simulink model "uz_mpc_6ph"  (R2021a)
settings: Solver=FixedStepDiscrete  StartTime=0.0  StopTime=3*1/f  RelTol=1e-3
values from neighbouring files (symbols this model uses):
  A = 1.0    (= 1)    [uz_6ph_pu_vsd_voltages_init.m]    (also in uz_mpc_6ph_init.m; uz_mpc_6ph_state_machine_init.m = 0.1)
  f = n_rpm/60.0*p    (= 250)    [uz_6ph_pu_vsd_voltages_init.m]    (also in uz_mpc_6ph_init.m; uz_mpc_6ph_state_machine_init.m = 83.3333333333)
  IB = sqrt(2)*IR    [uz_6ph_pu_vsd_voltages_init.m]    (also in uz_mpc_6ph_init.m; uz_mpc_6ph_state_machine_init.m)
  id_ref = 0.0    (= 0)    [uz_6ph_pu_vsd_voltages_init.m]    (also in uz_mpc_6ph_init.m; uz_mpc_6ph_state_machine_init.m)
  iq_ref = -10.0    (= -10)    [uz_6ph_pu_vsd_voltages_init.m]    (also in uz_mpc_6ph_init.m; uz_mpc_6ph_state_machine_init.m = 5)
  ix_ref = 0.0    (= 0)    [uz_6ph_pu_vsd_voltages_init.m]    (also in uz_mpc_6ph_init.m; uz_mpc_6ph_state_machine_init.m)
  iy_ref = 0.0    (= 0)    [uz_6ph_pu_vsd_voltages_init.m]    (also in uz_mpc_6ph_init.m; uz_mpc_6ph_state_machine_init.m)
  Ld_minus_Lq_over_LB = (Ld-Lq)/LB    [uz_6ph_pu_vsd_voltages_init.m]    (also in uz_mpc_6ph_init.m; uz_mpc_6ph_state_machine_init.m)
  Ld_over_LB = Ld/LB    [uz_6ph_pu_vsd_voltages_init.m]    (also in uz_mpc_6ph_init.m; uz_mpc_6ph_state_machine_init.m)
  Lq_over_LB = Lq/LB    [uz_6ph_pu_vsd_voltages_init.m]    (also in uz_mpc_6ph_init.m; uz_mpc_6ph_state_machine_init.m)
  omega_m = n_rpm*pi/30    (= 314.159265359)    [uz_6ph_pu_vsd_voltages_init.m]    (also in uz_mpc_6ph_init.m; uz_mpc_6ph_state_machine_init.m = 104.71975512)
  omegaB = nR*2*pi()/60*p    [uz_6ph_pu_vsd_voltages_init.m]    (also in uz_mpc_6ph_init.m; uz_mpc_6ph_state_machine_init.m)
  psi_pm_over_psiB = psi_pm/psiB    [uz_6ph_pu_vsd_voltages_init.m]    (also in uz_mpc_6ph_init.m; uz_mpc_6ph_state_machine_init.m)
  Rs_over_ZB = Rs/ZB    [uz_6ph_pu_vsd_voltages_init.m]    (also in uz_mpc_6ph_init.m; uz_mpc_6ph_state_machine_init.m)
  t_ADC = 1/f_ADC    (= 1e-05)    [uz_6ph_pu_vsd_voltages_init.m]    (also in uz_mpc_6ph_init.m; uz_mpc_6ph_state_machine_init.m; uz_typeconv_init.m)
  Ts_times_ZB_over_Ld = Ts*ZB/Ld    [uz_6ph_pu_vsd_voltages_init.m]    (also in uz_mpc_6ph_init.m; uz_mpc_6ph_state_machine_init.m)
  Ts_times_ZB_over_Lq = Ts*ZB/Lq    [uz_6ph_pu_vsd_voltages_init.m]    (also in uz_mpc_6ph_init.m; uz_mpc_6ph_state_machine_init.m)
  Ts_times_ZB_over_Lx = Ts*ZB/Lx    [uz_6ph_pu_vsd_voltages_init.m]    (also in uz_mpc_6ph_init.m; uz_mpc_6ph_state_machine_init.m)
  Ts_times_ZB_over_Ly = Ts*ZB/Ly    [uz_6ph_pu_vsd_voltages_init.m]    (also in uz_mpc_6ph_init.m; uz_mpc_6ph_state_machine_init.m)
  v_dc = 565.0    (= 565)    [uz_6ph_pu_vsd_voltages_init.m]    (also in uz_mpc_6ph_init.m; uz_mpc_6ph_state_machine_init.m)
  VB = sqrt(2/3)*VR    [uz_6ph_pu_vsd_voltages_init.m]    (also in uz_mpc_6ph_init.m; uz_mpc_6ph_state_machine_init.m)
libraries: fl_lib x7, nesl_utility x7, simulink x4, ee_lib x2, hdlsllib x1
(part 2 of 2)

== matlab function uz_mpc_6ph/error_calculation ==
  settings: fimath=fimath('RoundingMethod', 'Floor','OverflowAction', 'Wrap','ProductMode', 'FullPrecision', 'SumMode', 'FullPrecision')
  data: id_ref_pu input; e_id_pu output; iq_ref_pu input; ix_ref_pu input; iy_ref_pu input; id_pred_pu input; iq_pred_pu input; ix_pred_pu input; iy_pred_pu input; max_current_pu input; G input; e_iq_pu output; e_ix_pu output; e_iy_pu output; delta_u output; index_prev input
function [e_id_pu, e_iq_pu, e_ix_pu, e_iy_pu, delta_u] = error_calculation(id_ref_pu,iq_ref_pu,ix_ref_pu,iy_ref_pu,id_pred_pu,iq_pred_pu,ix_pred_pu,iy_pred_pu,max_current_pu,G, index_prev)

num_switching_states = 64;

fm = fimath();
id_ref_pu = fi(id_ref_pu,1,18,15,fm);
iq_ref_pu = fi(iq_ref_pu,1,18,15,fm);
ix_ref_pu = fi(ix_ref_pu,1,18,15,fm);
iy_ref_pu = fi(iy_ref_pu,1,18,15,fm);

id_pred_pu = fi(zeros(num_switching_states,1),1,27,24,fm);
iq_pred_pu = fi(zeros(num_switching_states,1),1,27,24,fm);
ix_pred_pu = fi(zeros(num_switching_states,1),1,27,24,fm);
iy_pred_pu = fi(zeros(num_switching_states,1),1,27,24,fm);

max_current_pu = fi(max_current_pu,1,18,15,fm);

e_id_pu = fi(zeros(num_switching_states,1),1,18,15,fm);
e_iq_pu = fi(zeros(num_switching_states,1),1,18,15,fm);
e_ix_pu = fi(zeros(num_switching_states,1),1,18,15,fm);
e_iy_pu = fi(zeros(num_switching_states,1),1,18,15,fm);
d_u = fi(zeros(num_switching_states,6),0,18,0,fm);


for i=1:num_switching_states %(SZ+1) für die 4 Schalterstellungen im ersten Zeithorizont den Fehler berechnen
    e_id_pu(i) = (id_ref_pu-id_pred_pu(i))^2;
    e_iq_pu(i) = (iq_ref_pu-iq_pred_pu(i))^2;
    e_ix_pu(i) = (ix_ref_pu-ix_pred_pu(i))^2;
    e_iy_pu(i) = (iy_ref_pu-iy_pred_pu(i))^2;
    % check for current limit
    check_limit = fi(sqrt(id_pred_pu(i)^2+iq_pred_pu(i)^2+ix_pred_pu(i)^2+iy_pred_pu(i)^2),1,18,15,fm);
    if ( check_limit > max_current_pu)
        e_id_pu(i) = 3.99; % max value for Sfix18_En15
        e_iq_pu(i) = 3.99;
        e_ix_pu(i) = 3.99;
        e_iy_pu(i) = 3.99;
    end
    % calculate switching effort
    G_next = [G(i,1), G(i,3), G(i,5), G(i,7), G(i,9), G(i,11)];
    G_prev = [G(index_prev,1), G(index_prev,3), G(index_prev,5), G(index_prev,7), G(index_prev,9), G(index_prev,11)];
    d_u(i,:) = (G_prev -  G_next).^2;
end


delta_u = fi(sum(d_u,2),0,18,0,fm); % Summe jeder Zeile von d_u, um die Summe an Umschaltvorgängen zu erhalten
end

== matlab function uz_mpc_6ph/cost_function ==
  settings: fimath=fimath('RoundingMethod', 'Floor','OverflowAction', 'Wrap','ProductMode', 'FullPrecision', 'SumMode', 'FullPrecision')
  data: e_id_pu input; costs output; e_iq_pu input; e_ix_pu input; e_iy_pu input; delta_u input; lambda_d input; lambda_q input; lambda_x input; lambda_y input; lambda_u input
function costs = cost_function(e_id_pu,e_iq_pu,e_ix_pu,e_iy_pu,delta_u,lambda_d,lambda_q,lambda_x,lambda_y,lambda_u)

fm = fimath();
lambda_d = fi(lambda_d,0,18,17,fm);
lambda_q = fi(lambda_q,0,18,17,fm);
lambda_x = fi(lambda_x,0,18,17,fm);
lambda_y = fi(lambda_y,0,18,17,fm);
lambda_u = fi(lambda_u,0,18,17,fm);

% error could be worst case 4^2 for each current component + 12^2 for
% switching effort = 208. Fits into sfix27_En18
costs = fi(lambda_d * e_id_pu + lambda_q * e_iq_pu + lambda_x * e_ix_pu + lambda_y * e_iy_pu + lambda_u * delta_u,1,27,18,fm);

end

== matlab function uz_mpc_6ph/MATLAB Function ==
  settings: fimath=fimath('RoundingMethod', 'Floor','OverflowAction', 'Wrap','ProductMode', 'FullPrecision', 'SumMode', 'FullPrecision')
  data: costs input; id_pred_pu input; iq_pred_pu input; ix_pred_pu input; iy_pred_pu input; index output; id_pred_idx_pu output; iq_pred_idx_pu output; ix_pred_idx_pu output; iy_pred_idx_pu output; G input; Gates output
function [index, id_pred_idx_pu, iq_pred_idx_pu, ix_pred_idx_pu, iy_pred_idx_pu, Gates] = optimize_costs(costs, id_pred_pu, iq_pred_pu, ix_pred_pu,iy_pred_pu, G)

fm = fimath();
costs = fi(costs,1,27,18,fm);


[m, idx] = min(costs);
index = fi(idx,0,18,0,fm);
Gates = [G(index,1),G(index,2),G(index,3),G(index,4),G(index,5),G(index,6),...
         G(index,7),G(index,8),G(index,9),G(index,10),G(index,11),G(index,12)]; 
id_pred_idx_pu = id_pred_pu(index);
iq_pred_idx_pu = iq_pred_pu(index);
ix_pred_idx_pu = ix_pred_pu(index);
iy_pred_idx_pu = iy_pred_pu(index);

end

== matlab function uz_mpc_6ph/uz_mpc_current ==
  data: id_pu input fixdt_type_dq_currents; iq_pu input fixdt_type_dq_currents; ix_pu input fixdt_type_xy_currents; iy_pu input fixdt_type_xy_currents; angle_el input fixdt_type_angle; vd_pu input fixdt_type_sin_cos; vq_pu input fixdt_type_sin_cos; vx_pu input; vy_pu input; omega_pu input fixdt_type_speed; id_ref_pu input fixdt_type_dqxy_ref_currents; iq_ref_pu input fixdt_type_dqxy_ref_currents; ix_ref_pu input fixdt_type_dqxy_ref_currents; iy_ref_pu input fixdt_type_dqxy_ref_currents; v_DC_pu input fixdt_type_voltage; G output boolean; i_d_pred_pu output fixdt_type_dqxy_ref_currents; i_q_pred_pu output fixdt_type_dqxy_ref_currents; i_x_pred_pu output fixdt_type_dqxy_ref_currents; i_y_pred_pu output fixdt_type_dqxy_ref_currents; T_el_pred_pu output fixdt_type_dqxy_ref_currents; index output fixdt_type_polepairs; id_delay_pu output fixdt_type_dqxy_ref_currents; iq_delay_pu output fixdt_type_dqxy_ref_currents; Rs_over_ZB input fixdt_type_constants; Ts_times_ZB_over_Ld input fixdt_type_constants; Ts_times_ZB_over_Lq input fixdt_type_constants; Ts_times_ZB_over_Lx input fixdt_type_constants; Ts_times_ZB_over_Ly input fixdt_type_constants; Ld_over_LB input fixdt_type_constants; Lq_over_LB input fixdt_type_constants; Ld_minus_Lq_over_LB input fixdt_type_constants; psi_pm_over_psiB input fixdt_type_constants; polepairs input fixdt_type_polepairs; max_current_pu input fixdt_type_max_current; lambda_u input fixdt_type_lambda; lambda_d input fixdt_type_lambda; lambda_q input fixdt_type_lambda; lambda_x input fixdt_type_lambda; lambda_y input fixdt_type_lambda
function [G,i_d_pred_pu,i_q_pred_pu,i_x_pred_pu,i_y_pred_pu,T_el_pred_pu,index,id_delay_pu,iq_delay_pu] = myMPC(id_pu,iq_pu,ix_pu,iy_pu,angle_el,vd_pu,vq_pu,vx_pu,vy_pu,omega_pu, id_ref_pu,iq_ref_pu,ix_ref_pu,iy_ref_pu, v_DC_pu, Rs_over_ZB, Ts_times_ZB_over_Ld, Ts_times_ZB_over_Lq, Ts_times_ZB_over_Lx, Ts_times_ZB_over_Ly, Ld_over_LB, Lq_over_LB, Ld_minus_Lq_over_LB, psi_pm_over_psiB, polepairs, max_current_pu, lambda_u, lambda_d, lambda_q, lambda_x, lambda_y)

% previous index of switching states
persistent index_prev; 
    if isempty(index_prev)
        index_prev = 1;
    end
    
    
    
    
    
    num_switching_states=64;   %Schalterzustände
    ui16_n=1;    %Position in der Fehlermatrix


    persistent G_prev;
    
    if isempty(G_prev)
        G_prev = boolean([0 0 0 0 0 0]);
    end
    
    e_iq = zeros(num_switching_states,1);
    e_id = zeros(num_switching_states,1);
    e_ix = zeros(num_switching_states,1);
    e_iy = zeros(num_switching_states,1);
    delta_u = zeros(num_switching_states,6);
    




    %  V0 V1 V2 V3 V4 V5 V6 V7 V8 V9 V10 V11 V12 V13 V14 V15 V16 V17 V18 V19 V20 V21 V22 V23 V24 V25 V26 V27 V28 V29 V30 V31 V32 V33 V34 V35 V36 V37 V38 V39 V40 V41 V42 V43 V44 V45 V46 V47 V48 V49 V50 V51 V52 V53 V54 V55 V56 V57 V58 V59 V60 V61 V62 V63      (Spannungsvektor)
s1_v = [0; 1; 0; 1; 0; 1; 0; 1; 0; 1; 0; 1; 0; 1; 0; 1; 0; 1; 0; 1; 0; ...
        1; 0; 1; 0; 1; 0; 1; 0; 1; 0; 1; 0; 1; 0; 1; 0; 1; 0; 1; 0; 1; ...
        0; 1; 0; 1; 0; 1; 0; 1; 0; 1; 0; 1; 0; 1; 0; 1; 0; 1; 0; 1; 0; ...
        1];

s2_v = [1; 0; 1; 0; 1; 0; 1; 0; 1; 0; 1; 0; 1; 0; 1; 0; 1; 0; 1; 0; 1; ...
        0; 1; 0; 1; 0; 1; 0; 1; 0; 1; 0; 1; 0; 1; 0; 1; 0; 1; 0; 1; 0; ...
        1; 0; 1; 0; 1; 0; 1; 0; 1; 0; 1; 0; 1; 0; 1; 0; 1; 0; 1; 0; 1; ...
        0];

s3_v = [0; 0; 1; 1; 0; 0; 1; 1; 0; 0; 1; 1; 0; 0; 1; 1; 0; 0; 1; 1; 0; ...
        0; 1; 1; 0; 0; 1; 1; 0; 0; 1; 1; 0; 0; 1; 1; 0; 0; 1; 1; 0; 0; ...
        1; 1; 0; 0; 1; 1; 0; 0; 1; 1; 0; 0; 1; 1; 0; 0; 1; 1; 0; 0; 1; ...
        1];

s4_v = [1; 1; 0; 0; 1; 1; 0; 0; 1; 1; 0; 0; 1; 1; 0; 0; 1; 1; 0; 0; 1; ...
        1; 0; 0; 1; 1; 0; 0; 1; 1; 0; 0; 1; 1; 0; 0; 1; 1; 0; 0; 1; 1; ...
        0; 0; 1; 1; 0; 0; 1; 1; 0; 0; 1; 1; 0; 0; 1; 1; 0; 0; 1; 1; 0; ...
        0];

s5_v = [0; 0; 0; 0; 1; 1; 1; 1; 0; 0; 0; 0; 1; 1; 1; 1; 0; 0; 0; 0; 1; ...
        1; 1; 1; 0; 0; 0; 0; 1; 1; 1; 1; 0; 0; 0; 0; 1; 1; 1; 1; 0; 0; ...
        0; 0; 1; 1; 1; 1; 0; 0; 0; 0; 1; 1; 1; 1; 0; 0; 0; 0; 1; 1; 1; ...
        1];

s6_v = [1; 1; 1; 1; 0; 0; 0; 0; 1; 1; 1; 1; 0; 0; 0; 0; 1; 1; 1; 1; 0; ...
        0; 0; 0; 1; 1; 1; 1; 0; 0; 0; 0; 1; 1; 1; 1; 0; 0; 0; 0; 1; 1; ...
        1; 1; 0; 0; 0; 0; 1; 1; 1; 1; 0; 0; 0; 0; 1; 1; 1; 1; 0; 0; 0; ...
        0];

s7_v = [0; 0; 0; 0; 0; 0; 0; 0; 1; 1; 1; 1; 1; 1; 1; 1; 0; 0; 0; 0; 0; ...
        0; 0; 0; 1; 1; 1; 1; 1; 1; 1; 1; 0; 0; 0; 0; 0; 0; 0; 0; 1; 1; ...
        1; 1; 1; 1; 1; 1; 0; 0; 0; 0; 0; 0; 0; 0; 1; 1; 1; 1; 1; 1; 1; ...
        1];

s8_v = [1; 1; 1; 1; 1; 1; 1; 1; 0; 0; 0; 0; 0; 0; 0; 0; 1; 1; 1; 1; 1; ...
        1; 1; 1; 0; 0; 0; 0; 0; 0; 0; 0; 1; 1; 1; 1; 1; 1; 1; 1; 0; 0; ...
        0; 0; 0; 0; 0; 0; 1; 1; 1; 1; 1; 1; 1; 1; 0; 0; 0; 0; 0; 0; 0; ...
        0];

s9_v = [0; 0; 0; 0; 0; 0; 0; 0; 0; 0; 0; 0; 0; 0; 0; 0; 1; 1; 1; 1; 1; ...
        1; 1; 1; 1; 1; 1; 1; 1; 1; 1; 1; 0; 0; 0; 0; 0; 0; 0; 0; 0; 0; ...
        0; 0; 0; 0; 0; 0; 1; 1; 1; 1; 1; 1; 1; 1; 1; 1; 1; 1; 1; 1; 1; ...
        1];

s10_v = [1; 1; 1; 1; 1; 1; 1; 1; 1; 1; 1; 1; 1; 1; 1; 1; 0; 0; 0; 0; 0; ...
         0; 0; 0; 0; 0; 0; 0; 0; 0; 0; 0; 1; 1; 1; 1; 1; 1; 1; 1; 1; 1; ...
         1; 1; 1; 1; 1; 1; 0; 0; 0; 0; 0; 0; 0; 0; 0; 0; 0; 0; 0; 0; 0; ...
         0];

s11_v = [0; 0; 0; 0; 0; 0; 0; 0; 0; 0; 0; 0; 0; 0; 0; 0; 0; 0; 0; 0; 0; ...
         0; 0; 0; 0; 0; 0; 0; 0; 0; 0; 0; 1; 1; 1; 1; 1; 1; 1; 1; 1; 1; ...
         1; 1; 1; 1; 1; 1; 1; 1; 1; 1; 1; 1; 1; 1; 1; 1; 1; 1; 1; 1; 1; ...
         1];

s12_v = [1; 1; 1; 1; 1; 1; 1; 1; 1; 1; 1; 1; 1; 1; 1; 1; 1; 1; 1; 1; 1; ...
         1; 1; 1; 1; 1; 1; 1; 1; 1; 1; 1; 0; 0; 0; 0; 0; 0; 0; 0; 0; 0; ...
         0; 0; 0; 0; 0; 0; 0; 0; 0; 0; 0; 0; 0; 0; 0; 0; 0; 0; 0; 0; 0; ...
         0];

                          

                
%Berechnung des aktuellen Modells zum Zeitpunkt (k+1), wenn die neue
%Schalterstellung angelegt wird. Dies geschieht anhand der alten,
%vorhergehenden Schalterstellung "idx_alt". Hierdurch wird die Delay-Time
%von einem diskreten Zeitschritt kompensiert!
    [id_delay_pu,iq_delay_pu,ix_delay_pu,iy_delay_pu] = predict_currents(vd_pu(index_prev),vq_pu(index_prev),vx_pu(index_prev),vy_pu(index_prev),id_pu,iq_pu,ix_pu,iy_pu,omega_pu,Ts_times_ZB_over_Ld,Ts_times_ZB_over_Lq,Ts_times_ZB_over_Lx,Ts_times_ZB_over_Ly,Rs_over_ZB,Ld_over_LB,Lq_over_LB,Ld_minus_Lq_over_LB,psi_pm_over_psiB,polepairs);

% id_delay_pu = id_delay_pu;
% iq_delay_pu = iq_delay_pu;
% hier könnte noch Algorithmik zur Eingrenzung der betrachteten
% Schalthandlungen stehen
    

%start Prädiktion %%%%%%%%%%%%%%%%%%%%%%%%%%%%%%%%%%%%%%%%%%%%%%%%%%%%%%%%%%%%%%%
    id_pu_nxt = zeros(num_switching_states, 1);
    iq_pu_nxt = zeros(num_switching_states, 1);
    ix_pu_nxt = zeros(num_switching_states, 1);
    iy_pu_nxt = zeros(num_switching_states, 1);
    T_el_pu_nxt = zeros(num_switching_states, 1);

        

    %Erster Zeithorizont
    for i = 1:num_switching_states
        [id_pu_nxt(i),iq_pu_nxt(i),ix_pu_nxt(i),iy_pu_nxt(i), T_el_pu_nxt(i)] = predict_currents(vd_pu(i),vq_pu(i),vx_pu(i),vy_pu(i),id_delay_pu,iq_delay_pu,ix_delay_pu,iy_delay_pu, omega_pu,Ts_times_ZB_over_Ld,Ts_times_ZB_over_Lq,Ts_times_ZB_over_Lx,Ts_times_ZB_over_Ly,Rs_over_ZB,Ld_over_LB,Lq_over_LB,Ld_minus_Lq_over_LB,psi_pm_over_psiB,polepairs);
    end
    
%end Prädiktion %%%%%%%%%%%%%%%%%%%%%%%%%%%%%%%%%%%%%%%%%%%%%%%%%%%%%%%%%%%



%start Optimierung des Gütekriteriums%%%%%%%%%%%%%%%%%%%%%%%%%%%%%%%%%%%%%%

           for i=1:num_switching_states %(SZ+1) für die 4 Schalterstellungen im ersten Zeithorizont den Fehler berechnen                  
                     e_iq(ui16_n) = (iq_ref_pu-fi(iq_pu_nxt(i),1,18,15))^2;                 
                     e_id(ui16_n) = (id_ref_pu-fi(id_pu_nxt(i),1,18,15))^2;
                     e_ix(ui16_n) = (ix_ref_pu-fi(ix_pu_nxt(i),1,18,15))^2;
                     e_iy(ui16_n) = (iy_ref_pu-fi(iy_pu_nxt(i),1,18,15))^2;
                     % Stromgrenze einhalten
%                      if ( (sqrt(id_pu_nxt(i)^2+iq_pu_nxt(i)^2+ix_pu_nxt(i)^2+iy_pu_nxt(i)^2)) > max_current_pu ) 
%                          e_iq(ui16_n) = e_iq(ui16_n)+10e4;%Wenn Stromgrenze überschritten, den Fehler auf
%                          %Maximalwertsetzen und disqualifizieren
%                          e_id(ui16_n) = e_id(ui16_n)+10e4;%Wenn Stromgrenze überschritten, den Fehler auf
%                          %Maximalwertsetzen und disqualifizieren
%                      end
                     %Schalten bestrafen
                     G_next = [s1_v(i), s3_v(i), s5_v(i), s7_v(i), s9_v(i), s11_v(i)];
                     delta_u(ui16_n,:) = (G_prev -  G_next).^2;
                    
%                 end
                ui16_n = ui16_n+1; %Hochzählen des Drehzahlfehlervektors
           end
           
           
           delta_u = sum(delta_u,2); % Summe jeder Zeile von d_u, um die Summe an Umschaltvorgängen zu erhalten
            
    cost_function = fi(e_id,1,18,15)*lambda_d + fi(e_iq,1,18,15)*lambda_q+fi(e_ix,1,18,15)*lambda_x+fi(e_iy,1,18,15)*lambda_y + fi(delta_u,1,18,15)*lambda_u; %Summe aller Fehler bildet die Zielfunktion 
    [m, ui8_idx] = min(cost_function); %Suche nach dem Minimum der Zielfunktion 

    index = uint32(ui8_idx);
    
%end Optimierung des Gütekriteriums%%%%%%%%%%%%%%%%%%%%%%%%%%%%%%%%%%%%%%%%

    ss_v = [
           s1_v(ui8_idx);
           s2_v(ui8_idx);
           s3_v(ui8_idx);  
           s4_v(ui8_idx); 
           s5_v(ui8_idx);
           s6_v(ui8_idx);
           s7_v(ui8_idx);
           s8_v(ui8_idx);
           s9_v(ui8_idx);
           s10_v(ui8_idx);
           s11_v(ui8_idx);
           s12_v(ui8_idx);
           ]; 
    G_prev = boolean([ss_v(1), ss_v(3), ss_v(5), ss_v(7), ss_v(9), ss_v(11)]);
    G = G_prev;
    index_prev = ui8_idx;          %Schalterstellung des vorherigen Schritts merken
%     d_theta_alt = theta;      %Winkel des vorherigen Schritts merken
    
    i_d_pred_pu = fi(id_pu_nxt(ui8_idx),1,18,15);
    i_q_pred_pu = fi(iq_pu_nxt(ui8_idx),1,18,15);
    i_x_pred_pu = fi(ix_pu_nxt(ui8_idx),1,18,15);
    i_y_pred_pu = fi(iy_pu_nxt(ui8_idx),1,18,15);
    T_el_pred_pu = fi(T_el_pu_nxt(ui8_idx),1,18,15);

end




function [id_pred_pu,iq_pred_pu,ix_pred_pu,iy_pred_pu, T_el_pred_pu] = predict_currents(vd_pu,vq_pu,vx_pu,vy_pu,id_k_pu,iq_k_pu,ix_k_pu,iy_k_pu,...
                                                                                        omega_m_pu,Ts_times_ZB_over_Ld,Ts_times_ZB_over_Lq,...
                                                                                        Ts_times_ZB_over_Lx,Ts_times_ZB_over_Ly,Rs_over_ZB,Ld_over_LB,...
                                                                                        Lq_over_LB,Ld_minus_Lq_over_LB,psi_pm_over_psiB,polepairs)
                                                                                  
    %Prediction d-current
    id_pred_pu = fi(Ts_times_ZB_over_Ld *(vd_pu - Rs_over_ZB * id_k_pu + iq_k_pu * Lq_over_LB * omega_m_pu * polepairs) + id_k_pu,1,18,15);
    
    %Prediction q-current
    iq_pred_pu = fi(Ts_times_ZB_over_Lq *(vq_pu - Rs_over_ZB * iq_k_pu - omega_m_pu * Ld_over_LB * id_k_pu - omega_m_pu * polepairs * psi_pm_over_psiB) + iq_k_pu,1,18,15);
       
    %Prediction x-current
    ix_pred_pu = fi(Ts_times_ZB_over_Lx *(vx_pu - Rs_over_ZB* ix_k_pu) + ix_k_pu,1,18,15);
   
    %Prediction y-current
    iy_pred_pu = fi(Ts_times_ZB_over_Ly *(vy_pu - Rs_over_ZB * iy_k_pu) + iy_k_pu,1,18,15);
    
    %Prediction air-gap torque
%     T_el_pred_pu = 3 * (psi_pm_over_psiB*iq_pred_pu + Ld_minus_Lq_over_LB *id_pred_pu*iq_pred_pu);
    T_el_pred_pu = 0;

end

== matlab function uz_mpc_6ph/uz_6ph_pu_voltages_vsd/finite_control_set ==
  data: v_DC_pu input; sin_angle input; pu_ud output; pu_uq output; pu_ux output; pu_uy output; cos_angle input
function [pu_ud,pu_uq,pu_ux,pu_uy] = voltage_space_vectors(v_DC_pu, sin_angle, cos_angle)
                          
% u_d-voltages
vd_pu = v_DC_pu * fi([0.000000*cos_angle + 0.000000*sin_angle;
0.333333*cos_angle + -0.000000*sin_angle;
-0.166667*cos_angle + 0.288675*sin_angle;
0.166667*cos_angle + 0.288675*sin_angle;
-0.166667*cos_angle + -0.288675*sin_angle;
0.166667*cos_angle + -0.288675*sin_angle;
-0.333333*cos_angle + 0.000000*sin_angle;
0.000000*cos_angle + 0.000000*sin_angle;
0.288675*cos_angle + 0.166667*sin_angle;
0.622008*cos_angle + 0.166667*sin_angle;
0.122008*cos_angle + 0.455342*sin_angle;
0.455342*cos_angle + 0.455342*sin_angle;
0.122008*cos_angle + -0.122008*sin_angle;
0.455342*cos_angle + -0.122008*sin_angle;
-0.044658*cos_angle + 0.166667*sin_angle;
0.288675*cos_angle + 0.166667*sin_angle;
-0.288675*cos_angle + 0.166667*sin_angle;
0.044658*cos_angle + 0.166667*sin_angle;
-0.455342*cos_angle + 0.455342*sin_angle;
-0.122008*cos_angle + 0.455342*sin_angle;
-0.455342*cos_angle + -0.122008*sin_angle;
-0.122008*cos_angle + -0.122008*sin_angle;
-0.622008*cos_angle + 0.166667*sin_angle;
-0.288675*cos_angle + 0.166667*sin_angle;
0.000000*cos_angle + 0.333333*sin_angle;
0.333333*cos_angle + 0.333333*sin_angle;
-0.166667*cos_angle + 0.622008*sin_angle;
0.166667*cos_angle + 0.622008*sin_angle;
-0.166667*cos_angle + 0.044658*sin_angle;
0.166667*cos_angle + 0.044658*sin_angle;
-0.333333*cos_angle + 0.333333*sin_angle;
0.000000*cos_angle + 0.333333*sin_angle;
-0.000000*cos_angle + -0.333333*sin_angle;
0.333333*cos_angle + -0.333333*sin_angle;
-0.166667*cos_angle + -0.044658*sin_angle;
0.166667*cos_angle + -0.044658*sin_angle;
-0.166667*cos_angle + -0.622008*sin_angle;
0.166667*cos_angle + -0.622008*sin_angle;
-0.333333*cos_angle + -0.333333*sin_angle;
-0.000000*cos_angle + -0.333333*sin_angle;
0.288675*cos_angle + -0.166667*sin_angle;
0.622008*cos_angle + -0.166667*sin_angle;
0.122008*cos_angle + 0.122008*sin_angle;
0.455342*cos_angle + 0.122008*sin_angle;
0.122008*cos_angle + -0.455342*sin_angle;
0.455342*cos_angle + -0.455342*sin_angle;
-0.044658*cos_angle + -0.166667*sin_angle;
0.288675*cos_angle + -0.166667*sin_angle;
-0.288675*cos_angle + -0.166667*sin_angle;
0.044658*cos_angle + -0.166667*sin_angle;
-0.455342*cos_angle + 0.122008*sin_angle;
-0.122008*cos_angle + 0.122008*sin_angle;
-0.455342*cos_angle + -0.455342*sin_angle;
-0.122008*cos_angle + -0.455342*sin_angle;
-0.622008*cos_angle + -0.166667*sin_angle;
-0.288675*cos_angle + -0.166667*sin_angle;
0.000000*cos_angle + 0.000000*sin_angle;
0.333333*cos_angle + -0.000000*sin_angle;
-0.166667*cos_angle + 0.288675*sin_angle;
0.166667*cos_angle + 0.288675*sin_angle;
-0.166667*cos_angle + -0.288675*sin_angle;
0.166667*cos_angle + -0.288675*sin_angle;
-0.333333*cos_angle + 0.000000*sin_angle;
0.000000*cos_angle + 0.000000*sin_angle],1,18,15);

% u_q-voltages
vq_pu = v_DC_pu * fi([0.000000*-sin_angle + 0.000000*cos_angle;
0.333333*-sin_angle + -0.000000*cos_angle;
-0.166667*-sin_angle + 0.288675*cos_angle;
0.166667*-sin_angle + 0.288675*cos_angle;
-0.166667*-sin_angle + -0.288675*cos_angle;
0.166667*-sin_angle + -0.288675*cos_angle;
-0.333333*-sin_angle + 0.000000*cos_angle;
0.000000*-sin_angle + 0.000000*cos_angle;
0.288675*-sin_angle + 0.166667*cos_angle;
0.622008*-sin_angle + 0.166667*cos_angle;
0.122008*-sin_angle + 0.455342*cos_angle;
0.455342*-sin_angle + 0.455342*cos_angle;
0.122008*-sin_angle + -0.122008*cos_angle;
0.455342*-sin_angle + -0.122008*cos_angle;
-0.044658*-sin_angle + 0.166667*cos_angle;
0.288675*-sin_angle + 0.166667*cos_angle;
-0.288675*-sin_angle + 0.166667*cos_angle;
0.044658*-sin_angle + 0.166667*cos_angle;
-0.455342*-sin_angle + 0.455342*cos_angle;
-0.122008*-sin_angle + 0.455342*cos_angle;
-0.455342*-sin_angle + -0.122008*cos_angle;
-0.122008*-sin_angle + -0.122008*cos_angle;
-0.622008*-sin_angle + 0.166667*cos_angle;
-0.288675*-sin_angle + 0.166667*cos_angle;
0.000000*-sin_angle + 0.333333*cos_angle;
0.333333*-sin_angle + 0.333333*cos_angle;
-0.166667*-sin_angle + 0.622008*cos_angle;
0.166667*-sin_angle + 0.622008*cos_angle;
-0.166667*-sin_angle + 0.044658*cos_angle;
0.166667*-sin_angle + 0.044658*cos_angle;
-0.333333*-sin_angle + 0.333333*cos_angle;
0.000000*-sin_angle + 0.333333*cos_angle;
-0.000000*-sin_angle + -0.333333*cos_angle;
0.333333*-sin_angle + -0.333333*cos_angle;
-0.166667*-sin_angle + -0.044658*cos_angle;
0.166667*-sin_angle + -0.044658*cos_angle;
-0.166667*-sin_angle + -0.622008*cos_angle;
0.166667*-sin_angle + -0.622008*cos_angle;
-0.333333*-sin_angle + -0.333333*cos_angle;
-0.000000*-sin_angle + -0.333333*cos_angle;
0.288675*-sin_angle + -0.166667*cos_angle;
0.622008*-sin_angle + -0.166667*cos_angle;
0.122008*-sin_angle + 0.122008*cos_angle;
0.455342*-sin_angle + 0.122008*cos_angle;
0.122008*-sin_angle + -0.455342*cos_angle;
0.455342*-sin_angle + -0.455342*cos_angle;
-0.044658*-sin_angle + -0.166667*cos_angle;
0.288675*-sin_angle + -0.166667*cos_angle;
-0.288675*-sin_angle + -0.166667*cos_angle;
0.044658*-sin_angle + -0.166667*cos_angle;
-0.455342*-sin_angle + 0.122008*cos_angle;
-0.122008*-sin_angle + 0.122008*cos_angle;
-0.455342*-sin_angle + -0.455342*cos_angle;
-0.122008*-sin_angle + -0.455342*cos_angle;
-0.622008*-sin_angle + -0.166667*cos_angle;
-0.288675*-sin_angle + -0.166667*cos_angle;
0.000000*-sin_angle + 0.000000*cos_angle;
0.333333*-sin_angle + -0.000000*cos_angle;
-0.166667*-sin_angle + 0.288675*cos_angle;
0.166667*-sin_angle + 0.288675*cos_angle;
-0.166667*-sin_angle + -0.288675*cos_angle;
0.166667*-sin_angle + -0.288675*cos_angle;
-0.333333*-sin_angle + 0.000000*cos_angle;
0.000000*-sin_angle + 0.000000*cos_angle],1,18,15);
     
% u_x-voltages
vx_pu = v_DC_pu * fi([0.000000;
0.333333;
-0.166667;
0.166667;
-0.166667;
0.166667;
-0.333333;
0.000000;
-0.288675;
0.044658;
-0.455342;
-0.122008;
-0.455342;
-0.122008;
-0.622008;
-0.288675;
0.288675;
0.622008;
0.122008;
0.455342;
0.122008;
0.455342;
-0.044658;
0.288675;
0.000000;
0.333333;
-0.166667;
0.166667;
-0.166667;
0.166667;
-0.333333;
0.000000;
-0.000000;
0.333333;
-0.166667;
0.166667;
-0.166667;
0.166667;
-0.333333;
-0.000000;
-0.288675;
0.044658;
-0.455342;
-0.122008;
-0.455342;
-0.122008;
-0.622008;
-0.288675;
0.288675;
0.622008;
0.122008;
0.455342;
0.122008;
0.455342;
-0.044658;
0.288675;
0.000000;
0.333333;
-0.166667;
0.166667;
-0.166667;
0.166667;
-0.333333;
0.000000],1,18,15);

% u_y-voltages
vy_pu = v_DC_pu * fi([0.000000;
-0.000000;
-0.288675;
-0.288675;
0.288675;
0.288675;
0.000000;
0.000000;
0.166667;
0.166667;
-0.122008;
-0.122008;
0.455342;
0.455342;
0.166667;
0.166667;
0.166667;
0.166667;
-0.122008;
-0.122008;
0.455342;
0.455342;
0.166667;
0.166667;
0.333333;
0.333333;
0.044658;
0.044658;
0.622008;
0.622008;
0.333333;
0.333333;
-0.333333;
-0.333333;
-0.622008;
-0.622008;
-0.044658;
-0.044658;
-0.333333;
-0.333333;
-0.166667;
-0.166667;
-0.455342;
-0.455342;
0.122008;
0.122008;
-0.166667;
-0.166667;
-0.166667;
-0.166667;
-0.455342;
-0.455342;
0.122008;
0.122008;
-0.166667;
-0.166667;
0.000000;
-0.000000;
-0.288675;
-0.288675;
0.288675;
0.288675;
0.000000;
0.000000],1,18,15);

pu_ud = fi(vd_pu,1,27,24);
pu_uq = fi(vq_pu,1,27,24);
pu_ux = fi(vx_pu,1,27,24);
pu_uy = fi(vy_pu,1,27,24);

== matlab function uz_mpc_6ph/FiniteControlSetSwitchingTable ==
  settings: fimath=fimath('RoundingMethod', 'Floor','OverflowAction', 'Wrap','ProductMode', 'FullPrecision', 'SumMode', 'FullPrecision')
  data: G output
function G  = switchingTable

% -------------------------------------------------------------------
%  Generated by MATLAB on 14-Oct-2020 14:52:37
%  MATLAB version: 9.4.0.813654 (R2018a)
% -------------------------------------------------------------------
                                         

s1_v = boolean([0; 1; 0; 1; 0; 1; 0; 1; 0; 1; 0; 1; 0; 1; 0; 1; 0; 1; 0; 1; 0; ...
        1; 0; 1; 0; 1; 0; 1; 0; 1; 0; 1; 0; 1; 0; 1; 0; 1; 0; 1; 0; 1; ...
        0; 1; 0; 1; 0; 1; 0; 1; 0; 1; 0; 1; 0; 1; 0; 1; 0; 1; 0; 1; 0; ...
        1]);


s2_v = boolean([1; 0; 1; 0; 1; 0; 1; 0; 1; 0; 1; 0; 1; 0; 1; 0; 1; 0; 1; 0; 1; ...
        0; 1; 0; 1; 0; 1; 0; 1; 0; 1; 0; 1; 0; 1; 0; 1; 0; 1; 0; 1; 0; ...
        1; 0; 1; 0; 1; 0; 1; 0; 1; 0; 1; 0; 1; 0; 1; 0; 1; 0; 1; 0; 1; ...
        0]);


s3_v = boolean([0; 0; 1; 1; 0; 0; 1; 1; 0; 0; 1; 1; 0; 0; 1; 1; 0; 0; 1; 1; 0; ...
        0; 1; 1; 0; 0; 1; 1; 0; 0; 1; 1; 0; 0; 1; 1; 0; 0; 1; 1; 0; 0; ...
        1; 1; 0; 0; 1; 1; 0; 0; 1; 1; 0; 0; 1; 1; 0; 0; 1; 1; 0; 0; 1; ...
        1]);


s4_v = boolean([1; 1; 0; 0; 1; 1; 0; 0; 1; 1; 0; 0; 1; 1; 0; 0; 1; 1; 0; 0; 1; ...
        1; 0; 0; 1; 1; 0; 0; 1; 1; 0; 0; 1; 1; 0; 0; 1; 1; 0; 0; 1; 1; ...
        0; 0; 1; 1; 0; 0; 1; 1; 0; 0; 1; 1; 0; 0; 1; 1; 0; 0; 1; 1; 0; ...
        0]);


s5_v = boolean([0; 0; 0; 0; 1; 1; 1; 1; 0; 0; 0; 0; 1; 1; 1; 1; 0; 0; 0; 0; 1; ...
        1; 1; 1; 0; 0; 0; 0; 1; 1; 1; 1; 0; 0; 0; 0; 1; 1; 1; 1; 0; 0; ...
        0; 0; 1; 1; 1; 1; 0; 0; 0; 0; 1; 1; 1; 1; 0; 0; 0; 0; 1; 1; 1; ...
        1]);


s6_v = boolean([1; 1; 1; 1; 0; 0; 0; 0; 1; 1; 1; 1; 0; 0; 0; 0; 1; 1; 1; 1; 0; ...
        0; 0; 0; 1; 1; 1; 1; 0; 0; 0; 0; 1; 1; 1; 1; 0; 0; 0; 0; 1; 1; ...
        1; 1; 0; 0; 0; 0; 1; 1; 1; 1; 0; 0; 0; 0; 1; 1; 1; 1; 0; 0; 0; ...
        0]);


s7_v = boolean([0; 0; 0; 0; 0; 0; 0; 0; 1; 1; 1; 1; 1; 1; 1; 1; 0; 0; 0; 0; 0; ...
        0; 0; 0; 1; 1; 1; 1; 1; 1; 1; 1; 0; 0; 0; 0; 0; 0; 0; 0; 1; 1; ...
        1; 1; 1; 1; 1; 1; 0; 0; 0; 0; 0; 0; 0; 0; 1; 1; 1; 1; 1; 1; 1; ...
        1]);


s8_v = boolean([1; 1; 1; 1; 1; 1; 1; 1; 0; 0; 0; 0; 0; 0; 0; 0; 1; 1; 1; 1; 1; ...
        1; 1; 1; 0; 0; 0; 0; 0; 0; 0; 0; 1; 1; 1; 1; 1; 1; 1; 1; 0; 0; ...
        0; 0; 0; 0; 0; 0; 1; 1; 1; 1; 1; 1; 1; 1; 0; 0; 0; 0; 0; 0; 0; ...
        0]);


s9_v = boolean([0; 0; 0; 0; 0; 0; 0; 0; 0; 0; 0; 0; 0; 0; 0; 0; 1; 1; 1; 1; 1; ...
        1; 1; 1; 1; 1; 1; 1; 1; 1; 1; 1; 0; 0; 0; 0; 0; 0; 0; 0; 0; 0; ...
        0; 0; 0; 0; 0; 0; 1; 1; 1; 1; 1; 1; 1; 1; 1; 1; 1; 1; 1; 1; 1; ...
        1]);


s10_v = boolean([1; 1; 1; 1; 1; 1; 1; 1; 1; 1; 1; 1; 1; 1; 1; 1; 0; 0; 0; 0; 0; ...
         0; 0; 0; 0; 0; 0; 0; 0; 0; 0; 0; 1; 1; 1; 1; 1; 1; 1; 1; 1; 1; ...
         1; 1; 1; 1; 1; 1; 0; 0; 0; 0; 0; 0; 0; 0; 0; 0; 0; 0; 0; 0; 0; ...
         0]);


s11_v = boolean([0; 0; 0; 0; 0; 0; 0; 0; 0; 0; 0; 0; 0; 0; 0; 0; 0; 0; 0; 0; 0; ...
         0; 0; 0; 0; 0; 0; 0; 0; 0; 0; 0; 1; 1; 1; 1; 1; 1; 1; 1; 1; 1; ...
         1; 1; 1; 1; 1; 1; 1; 1; 1; 1; 1; 1; 1; 1; 1; 1; 1; 1; 1; 1; 1; ...
         1]);


s12_v = boolean([1; 1; 1; 1; 1; 1; 1; 1; 1; 1; 1; 1; 1; 1; 1; 1; 1; 1; 1; 1; 1; ...
         1; 1; 1; 1; 1; 1; 1; 1; 1; 1; 1; 0; 0; 0; 0; 0; 0; 0; 0; 0; 0; ...
         0; 0; 0; 0; 0; 0; 0; 0; 0; 0; 0; 0; 0; 0; 0; 0; 0; 0; 0; 0; 0; ...
         0]);
     
G = [s1_v, s2_v, s3_v, s4_v, s5_v, s6_v, s7_v, s8_v, s9_v, s10_v, s11_v, s12_v];

== matlab function uz_mpc_6ph/delay_compensation ==
  settings: fimath=fimath('RoundingMethod', 'Floor','OverflowAction', 'Wrap','ProductMode', 'FullPrecision', 'SumMode', 'FullPrecision')
  data: vd_pu input; id_delay_pu output; vq_pu input; vx_pu input; vy_pu input; id_k_pu input; iq_k_pu input; ix_k_pu input; iy_k_pu input; omega_m_pu input; Ts_times_ZB_over_Ld input; Ts_times_ZB_over_Lq input; Ts_times_ZB_over_Lx input; Ts_times_ZB_over_Ly input; Rs_over_ZB input; Ld_over_LB input; Lq_over_LB input; psi_pm_over_psiB input; polepairs input; iq_delay_pu output; ix_delay_pu output; iy_delay_pu output; index input
function [id_delay_pu,iq_delay_pu,ix_delay_pu,iy_delay_pu] = predict_currents(vd_pu,vq_pu,vx_pu,vy_pu,id_k_pu,iq_k_pu,ix_k_pu,iy_k_pu,...
                                                                                        omega_m_pu,Ts_times_ZB_over_Ld,Ts_times_ZB_over_Lq,...
                                                                                        Ts_times_ZB_over_Lx,Ts_times_ZB_over_Ly,Rs_over_ZB,Ld_over_LB,...
                                                                                        Lq_over_LB,psi_pm_over_psiB,polepairs,index)                                                                     
    
    fm = fimath();
    vd_pu = fi(vd_pu,1,27,24,fm);
    vq_pu = fi(vq_pu,1,27,24,fm);
    vx_pu = fi(vx_pu,1,27,24,fm);
    vy_pu = fi(vy_pu,1,27,24,fm);
    
    id_k_pu = fi(id_k_pu,1,27,16,fm);
    iq_k_pu = fi(iq_k_pu,1,27,16,fm);
    ix_k_pu = fi(ix_k_pu,1,27,16,fm);
    iy_k_pu = fi(iy_k_pu,1,27,16,fm);
    
    omega_m_pu = fi(omega_m_pu,1,18,15,fm);
    
    Ts_times_ZB_over_Ld = fi(Ts_times_ZB_over_Ld,1,18,15,fm);
    Ts_times_ZB_over_Lq = fi(Ts_times_ZB_over_Lq,1,18,15,fm);
    Ts_times_ZB_over_Lx = fi(Ts_times_ZB_over_Lx,1,18,15,fm);
    Ts_times_ZB_over_Ly = fi(Ts_times_ZB_over_Ly,1,18,15,fm);
    Rs_over_ZB = fi(Rs_over_ZB,1,18,15,fm);
    Ld_over_LB = fi(Ld_over_LB,1,18,15,fm);
    Lq_over_LB = fi(Lq_over_LB,1,18,15,fm);
    psi_pm_over_psiB = fi(psi_pm_over_psiB,1,18,15,fm);
    polepairs = fi(polepairs,0,18,0,fm);
    index = fi(index,0,18,0,fm);
    
    %Prediction d-current
    id_delay_pu = fi(Ts_times_ZB_over_Ld *(vd_pu(index) - Rs_over_ZB * id_k_pu + iq_k_pu * Lq_over_LB * omega_m_pu * polepairs) + id_k_pu,1,27,24);
    
    %Prediction q-current
    iq_delay_pu = fi(Ts_times_ZB_over_Lq *(vq_pu(index) - Rs_over_ZB * iq_k_pu - omega_m_pu * polepairs * Ld_over_LB * id_k_pu - omega_m_pu * polepairs * psi_pm_over_psiB) + iq_k_pu,1,27,24);
       
    %Prediction x-current
    ix_delay_pu = fi(Ts_times_ZB_over_Lx *(vx_pu(index) - Rs_over_ZB* ix_k_pu) + ix_k_pu,1,27,24);
   
    %Prediction y-current
    iy_delay_pu = fi(Ts_times_ZB_over_Ly *(vy_pu(index) - Rs_over_ZB * iy_k_pu) + iy_k_pu,1,27,24);
  
end
